simulink model "quadcopter_kalman_test"  (R2015b)
settings: Solver=VariableStepAuto  StartTime=0.0  StopTime=50  RelTol=1e-3
undefined symbols (not defined in the file or in its folder): Do, euleranglelim, Io, N, omegalim, Po, seed
libraries: vrlib x2, simulink x2
settings Model: Creator=Daniel  LastModifiedBy=mgreiff
settings SolverCC: AlgebraicLoopSolver=LineSearch

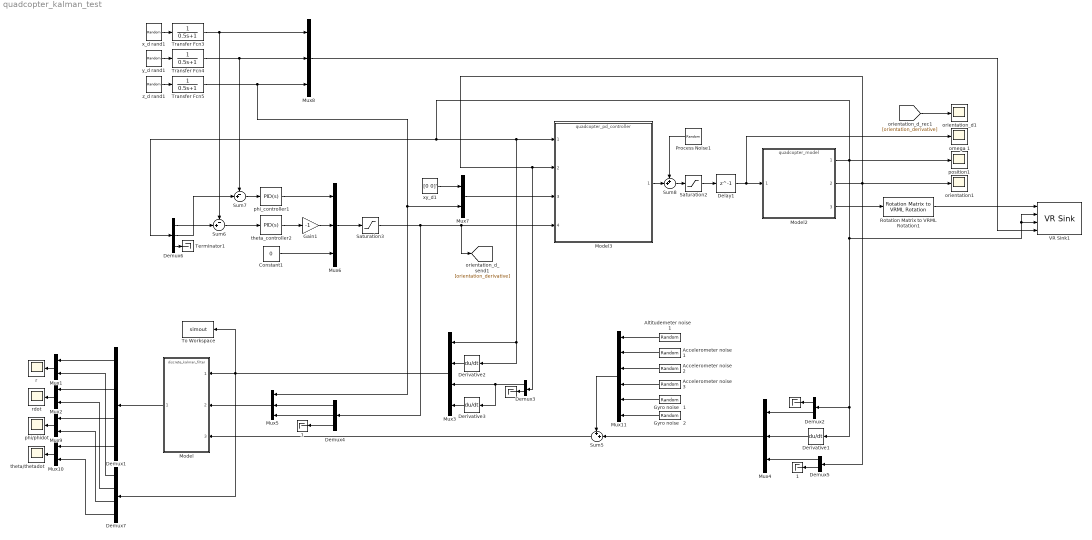
== system quadcopter_kalman_test ==
  "       " : Terminator
  "          " : Terminator
  "           1" : Terminator
  "          1" : Terminator
  Accelerometer noise  1 : RandomNumber  Variance=0.001  Seed=13  SampleTime=0.01
  Accelerometer noise  2 : RandomNumber  Variance=0.001  Seed=14  SampleTime=0.01
  Accelerometer noise  3 : RandomNumber  Variance=0.001  Seed=15  SampleTime=0.01
  Altitudemeter noise    1 : RandomNumber  Variance=0.01  Seed=12  SampleTime=0.01
  Constant1 : Constant  Value=0
  Delay1 : Delay  DelayLength=1  InitialCondition=0  SampleTime=0.01
  Demux1 : Demux  Outputs=[3,3,2,2]
  Demux2 : Demux  Outputs=[2,1]
  Demux3 : Demux  Outputs=[2,1]
  Demux4 : Demux  Outputs=[1,1,1]
  Demux5 : Demux  Outputs=[2,1]
  Demux6 : Demux  Outputs=3
  Demux7 : Demux  Outputs=[3,3,2,2]
  Derivative1 : Derivative
  Derivative2 : Derivative
  Derivative3 : Derivative
  Gain1 : Gain  Gain=-1
  Gyro noise   1 : RandomNumber  Variance=0.001  Seed=16  SampleTime=0.01
  Gyro noise   2 : RandomNumber  Variance=0.001  Seed=17  SampleTime=0.01
  Model : ModelReference  ModelNameDialog=discrete_kalman_filter.slx  SimulationMode=Normal  ModelReferenceVersion=1.56  CopyOfModelName=discrete_kalman_filter.slx
  Model2 : ModelReference  ModelNameDialog=quadcopter_model.mdl  SimulationMode=Normal  ModelReferenceVersion=1.114  CopyOfModelName=quadcopter_model.mdl
  Model3 : ModelReference  ModelNameDialog=quadcopter_pd_controller.mdl  SimulationMode=Normal  ModelReferenceVersion=1.60  CopyOfModelName=quadcopter_pd_controller.mdl
  Mux{1..2,7,9..10} (5 alike) : Mux  Inputs=2
  Mux11 : Mux  Inputs=6
  Mux3 : Mux  Inputs=[3,3,2,2]
  Mux4 : Mux  Inputs=3
  Mux5 : Mux  Inputs=[1,1,1]
  Mux6 : Mux  Inputs=3
  Mux8 : Mux  Inputs=3
  Process Noise1 : RandomNumber  Mean=[0 0 0 0]'  Variance=0.1  Seed=20  SampleTime=0.01
  Rotation Matrix to VRML Rotation1 : vrlib/Utilities/Rotation Matrix to VRML Rotation  maxzero=1e-12
  Saturation2 : Saturate  UpperLimit=omegalim(2)  LowerLimit=omegalim(1)
  Saturation3 : Saturate  UpperLimit=euleranglelim(2)  LowerLimit=euleranglelim(1)
  Sum5 : Sum  Inputs=++|
  Sum6 : Sum  Inputs=-+|
  Sum7 : Sum  Inputs=-+|
  Sum8 : Sum  Inputs=++|
  Terminator1 : Terminator
  To Workspace : ToWorkspace  VariableName=simout  SaveFormat=Timeseries  SampleTime=-1
  Transfer Fcn3 : TransferFcn  Denominator=[0.5 1]
  Transfer Fcn4 : TransferFcn  Denominator=[0.5 1]
  Transfer Fcn5 : TransferFcn  Denominator=[0.5 1]
  VR Sink1 : vrlib/VR Sink  InstantiateOnLoad=on  SampleTime=0.05  ViewEnable=on  RemoteChange=off  RemoteView=off  FieldsWritten=copter.rotation.4.1.1.double#copter.translation.3.1.1.double#vp.translation.3.1.1.double#target.translation.3.1.1.double  WorldFileName=copter_world.wrl  WorldDescription=quadcopter_world  AutoView=on  VideoDimensions=[]  AllowVariableSize=off
  omega 1 : Scope
  orientation1 : Scope
  orientation_d1 : Scope
  phi/phidot : Scope
  phi_controller1 : simulink/Continuous/PID Controller  Controller=PID  TimeDomain=Continuous-time  SampleTime=-1  IntegratorMethod=Forward Euler  FilterMethod=Forward Euler  Form=Parallel  UseFilter=on  ControllerParametersSource=internal  P=Po  I=Io  D=Do  N=N  InitialConditionSource=internal  InitialConditionForIntegrator=0  InitialConditionForFilter=0  ExternalReset=none  LimitOutput=off  UpperSaturationLimit=inf  LowerSaturationLimit=-inf  LinearizeAsGain=on  AntiWindupMode=none  Kb=1  TrackingMode=off  Kt=1  PParamMin=[]  PParamMax=[]  IParamMin=[]  IParamMax=[]  DParamMin=[]  DParamMax=[]  NParamMin=[]  NParamMax=[]  KbParamMin=[]  KbParamMax=[]  KtParamMin=[]  KtParamMax=[]  POutMin=[]  POutMax=[]  IOutMin=[]  IOutMax=[]  DOutMin=[]  DOutMax=[]  NOutMin=[]  NOutMax=[]  KbOutMin=[]  KbOutMax=[]  KtOutMin=[]  KtOutMax=[]  IntegratorOutMin=[]  IntegratorOutMax=[]  FilterOutMin=[]  FilterOutMax=[]  SumOutMin=[]  SumOutMax=[]  SumI1OutMin=[]  SumI1OutMax=[]  SumI2OutMin=[]  SumI2OutMax=[]  SumI3OutMin=[]  SumI3OutMax=[]  SumDOutMin=[]  SumDOutMax=[]  SaturationOutMin=[]  SaturationOutMax=[]  IntegratorContinuousStateAttributes=''  IntegratorStateMustResolveToSignalObject=off  IntegratorRTWStateStorageClass=Auto  FilterContinuousStateAttributes=''  FilterStateMustResolveToSignalObject=off  FilterRTWStateStorageClass=Auto  DifferentiatorICPrevScaledInput=0  DifferentiatorOutMin=[]  DifferentiatorOutMax=[]
  position1 : Scope
  r : Scope
  rdot : Scope
  theta/thetadot : Scope
  theta_controller2 : simulink/Continuous/PID Controller  Controller=PID  TimeDomain=Continuous-time  SampleTime=-1  IntegratorMethod=Forward Euler  FilterMethod=Forward Euler  Form=Parallel  UseFilter=on  ControllerParametersSource=internal  P=Po  I=Io  D=Do  N=N  InitialConditionSource=internal  InitialConditionForIntegrator=0  InitialConditionForFilter=0  ExternalReset=none  LimitOutput=off  UpperSaturationLimit=inf  LowerSaturationLimit=-inf  LinearizeAsGain=on  AntiWindupMode=none  Kb=1  TrackingMode=off  Kt=1  PParamMin=[]  PParamMax=[]  IParamMin=[]  IParamMax=[]  DParamMin=[]  DParamMax=[]  NParamMin=[]  NParamMax=[]  KbParamMin=[]  KbParamMax=[]  KtParamMin=[]  KtParamMax=[]  POutMin=[]  POutMax=[]  IOutMin=[]  IOutMax=[]  DOutMin=[]  DOutMax=[]  NOutMin=[]  NOutMax=[]  KbOutMin=[]  KbOutMax=[]  KtOutMin=[]  KtOutMax=[]  IntegratorOutMin=[]  IntegratorOutMax=[]  FilterOutMin=[]  FilterOutMax=[]  SumOutMin=[]  SumOutMax=[]  SumI1OutMin=[]  SumI1OutMax=[]  SumI2OutMin=[]  SumI2OutMax=[]  SumI3OutMin=[]  SumI3OutMax=[]  SumDOutMin=[]  SumDOutMax=[]  SaturationOutMin=[]  SaturationOutMax=[]  IntegratorContinuousStateAttributes=''  IntegratorStateMustResolveToSignalObject=off  IntegratorRTWStateStorageClass=Auto  FilterContinuousStateAttributes=''  FilterStateMustResolveToSignalObject=off  FilterRTWStateStorageClass=Auto  DifferentiatorICPrevScaledInput=0  DifferentiatorOutMin=[]  DifferentiatorOutMax=[]
  x_d rand1 : UniformRandomNumber  Minimum=-30  Maximum=30  Seed=0+seed  SampleTime=10
  xy_d1 : Constant  Value=[0 0]'
  y_d rand1 : UniformRandomNumber  Minimum=-30  Maximum=30  Seed=1+seed  SampleTime=10
  z_d rand1 : UniformRandomNumber  Minimum=0  Maximum=15  Seed=2+seed  SampleTime=10
  wires:
  Saturation2/1 -> Delay1/1
  Model2/3 -> Rotation Matrix to VRML Rotation1/1
  Constant1/1 -> Mux6/3
  theta_controller2/1 -> Gain1/1
  phi_controller1/1 -> Mux6/1
  Demux6/3 -> Terminator1/1
  x_d rand1/1 -> Transfer Fcn3/1
  y_d rand1/1 -> Transfer Fcn4/1
  Gain1/1 -> Mux6/2
  Mux6/1 -> Saturation3/1
  Demux6/2 -> Sum7/2
  Demux6/1 -> Sum6/2
  xy_d1/1 -> Mux7/1
  z_d rand1/1 -> Transfer Fcn5/1
  Rotation Matrix to VRML Rotation1/1 -> VR Sink1/1
  Mux8/1 -> VR Sink1/4
  Transfer Fcn3/1 -> Sum6/1, Mux8/1
  Transfer Fcn4/1 -> Sum7/1, Mux8/2
  Sum8/1 -> Saturation2/1
  Delay1/1 -> omega 1/1, Model2/1
  [orientation_derivative] -> orientation_d1/1
  Model3/1 -> Sum8/2
  Model2/1 -> Mux3/1, Derivative2/1, Model3/1, Demux6/1, Derivative1/1, Demux2/1, VR Sink1/2, VR Sink1/3, position1/1
  Sum6/1 -> theta_controller2/1
  Sum7/1 -> phi_controller1/1
  Saturation3/1 -> Demux4/1, [orientation_derivative], Model3/4
  Mux7/1 -> Model3/3
  Transfer Fcn5/1 -> Mux5/1, Mux7/2, Mux8/3
  Mux3/1 -> Model/1, Demux7/1, To Workspace/1
  Mux5/1 -> Model/2
  Demux2/1 -> "       "/1
  Demux3/2 -> "          "/1
  Model2/2 -> Demux5/1, Demux3/1, Model3/2, orientation1/1
  Demux5/2 -> "           1"/1
  Demux2/2 -> Mux4/1
  Derivative1/1 -> Mux4/2
  Demux5/1 -> Mux4/3
  Demux3/1 -> Derivative3/1, Mux3/3
  Mux1/1 -> r/1
  Mux2/1 -> rdot/1
  Mux9/1 -> phi/phidot/1
  Mux10/1 -> theta/thetadot/1
  Demux1/4 -> Mux10/1
  Demux1/3 -> Mux9/1
  Demux1/2 -> Mux2/1
  Demux1/1 -> Mux1/1
  Demux7/1 -> Mux1/2
  Demux7/2 -> Mux2/2
  Demux7/3 -> Mux9/2
  Demux7/4 -> Mux10/2
  Derivative2/1 -> Mux3/2
  Derivative3/1 -> Mux3/4
  Demux4/1 -> Mux5/2
  Demux4/3 -> "          1"/1
  Demux4/2 -> Mux5/3
  Altitudemeter noise    1/1 -> Mux11/1
  Accelerometer noise  1/1 -> Mux11/2
  Accelerometer noise  2/1 -> Mux11/3
  Accelerometer noise  3/1 -> Mux11/4
  Gyro noise   1/1 -> Mux11/5
  Gyro noise   2/1 -> Mux11/6
  Mux4/1 -> Sum5/2
  Mux11/1 -> Sum5/1
  Sum5/1 -> Model/3
  Process Noise1/1 -> Sum8/1
  Model/1 -> Demux1/1
